simulink model "four_channel_bilateral_teleoperation_sampled"  (R2020b)
settings: Solver=VariableStepAuto  StartTime=0.0  StopTime=4.0  RelTol=1e-3
values from neighbouring files (symbols this model uses):
  A = 1    [four_channel_bilateral_teleoperation_kalman_params.m]    (also in four_channel_bilateral_teleoperation_params.m; kalman_test.m = [1 Ts Ts^2/2; 0 1 Ts; 0 0 1]; recursive_estimation.m = [1 Ts Ts^2/2; 0 1 Ts; 0 0 1]; scattering_based_bi_teleop_pf_kalman_params.m)
  Be = 100    [four_channel_bilateral_teleoperation_architecture_params.m]    (also in four_channel_bilateral_teleoperation_kalman_params.m = 0; four_channel_bilateral_teleoperation_params.m = 0; scattering_based_bi_teleop_pf_kalman_params.m = 10; scattering_based_bi_teleop_pf_params.m = 10)
  Bh = 70    [four_channel_bilateral_teleoperation_architecture_params.m]    (also in four_channel_bilateral_teleoperation_kalman_params.m; four_channel_bilateral_teleoperation_params.m; scattering_based_bi_teleop_pf_kalman_params.m = 1.5; scattering_based_bi_teleop_pf_params.m = 1.5)
  Bm = 1    [four_channel_bilateral_teleoperation_architecture_params.m]    (also in four_channel_bilateral_teleoperation_kalman_params.m = 0.8; four_channel_bilateral_teleoperation_params.m = 0.8; scattering_based_bi_teleop_pf_kalman_params.m = 0; scattering_based_bi_teleop_pp_kalman_params.m = 15)
  Bs = 1    [four_channel_bilateral_teleoperation_architecture_params.m]    (also in four_channel_bilateral_teleoperation_kalman_params.m = 3.2; four_channel_bilateral_teleoperation_params.m = 3.2; scattering_based_bi_teleop_pf_kalman_params.m = 40; scattering_based_bi_teleop_pf_params.m = 3)
  Dh = 500    [four_channel_bilateral_teleoperation_kalman_params.m]    (also in four_channel_bilateral_teleoperation_params.m = 100; scattering_based_bi_teleop_pf_kalman_params.m = 0; scattering_based_bi_teleop_pf_params.m = 17; scattering_based_bi_teleop_pp_kalman_params.m = 0)
  Dm = 5    [four_channel_bilateral_teleoperation_architecture_params.m]    (also in four_channel_bilateral_teleoperation_kalman_params.m = 0; four_channel_bilateral_teleoperation_params.m = 0; scattering_based_bi_teleop_pf_kalman_params.m = 0; scattering_based_bi_teleop_pf_params.m = 0)
  Ds = 10    [four_channel_bilateral_teleoperation_architecture_params.m]    (also in four_channel_bilateral_teleoperation_kalman_params.m = 0; four_channel_bilateral_teleoperation_params.m = 0; scattering_based_bi_teleop_pf_kalman_params.m = 0; scattering_based_bi_teleop_pf_params.m = 0)
  Fc = 1    [four_channel_bilateral_teleoperation_kalman_params.m]    (also in four_channel_bilateral_teleoperation_params.m; kalman_test.m = 10; scattering_based_bi_teleop_pf_kalman_params.m = 0.1; scattering_based_bi_teleop_pf_params.m)
  Fip = 1    [four_channel_bilateral_teleoperation_kalman_params.m]    (also in four_channel_bilateral_teleoperation_params.m; scattering_based_bi_teleop_pf_kalman_params.m = 5; scattering_based_bi_teleop_pf_params.m; scattering_based_bi_teleop_pp_kalman_params.m = 5)
  Je = 0    [four_channel_bilateral_teleoperation_architecture_params.m]    (also in four_channel_bilateral_teleoperation_kalman_params.m; four_channel_bilateral_teleoperation_params.m; scattering_based_bi_teleop_pf_kalman_params.m; scattering_based_bi_teleop_pf_params.m)
  Jh = 0.5    [four_channel_bilateral_teleoperation_architecture_params.m]    (also in four_channel_bilateral_teleoperation_kalman_params.m; four_channel_bilateral_teleoperation_params.m; scattering_based_bi_teleop_pf_kalman_params.m = 0; scattering_based_bi_teleop_pf_params.m = 0.05)
  Ke = 200    [four_channel_bilateral_teleoperation_architecture_params.m]    (also in four_channel_bilateral_teleoperation_kalman_params.m = 50; four_channel_bilateral_teleoperation_params.m; scattering_based_bi_teleop_pf_kalman_params.m; scattering_based_bi_teleop_pf_params.m)
  Kh = 2000    [four_channel_bilateral_teleoperation_architecture_params.m]    (also in four_channel_bilateral_teleoperation_kalman_params.m; four_channel_bilateral_teleoperation_params.m; scattering_based_bi_teleop_pf_kalman_params.m = 1; scattering_based_bi_teleop_pf_params.m = 0)
  Km = 1    [four_channel_bilateral_teleoperation_architecture_params.m]    (also in four_channel_bilateral_teleoperation_kalman_params.m; four_channel_bilateral_teleoperation_params.m; scattering_based_bi_teleop_pf_kalman_params.m = 0; scattering_based_bi_teleop_pp_kalman_params.m = 10)
  Ks = 1    [four_channel_bilateral_teleoperation_architecture_params.m]    (also in four_channel_bilateral_teleoperation_kalman_params.m = 4; four_channel_bilateral_teleoperation_params.m = 4; scattering_based_bi_teleop_pf_kalman_params.m = 50; scattering_based_bi_teleop_pf_params.m = 110)
  Mm = 0.5    [four_channel_bilateral_teleoperation_architecture_params.m]    (also in four_channel_bilateral_teleoperation_kalman_params.m; four_channel_bilateral_teleoperation_params.m; scattering_based_bi_teleop_pf_kalman_params.m; scattering_based_bi_teleop_pf_params.m)
  Ms = 2    [four_channel_bilateral_teleoperation_architecture_params.m]    (also in four_channel_bilateral_teleoperation_kalman_params.m; four_channel_bilateral_teleoperation_params.m; scattering_based_bi_teleop_pf_kalman_params.m; scattering_based_bi_teleop_pf_params.m)
  Ph = 2000    [four_channel_bilateral_teleoperation_kalman_params.m]    (also in four_channel_bilateral_teleoperation_params.m = 20100; scattering_based_bi_teleop_pf_kalman_params.m = 5; scattering_based_bi_teleop_pf_params.m = 23; scattering_based_bi_teleop_pp_kalman_params.m = 6)
  Ts = 0.001    [four_channel_bilateral_teleoperation_kalman_params.m]    (also in four_channel_bilateral_teleoperation_params.m; kalman_test.m; recursive_estimation.m; scattering_based_bi_teleop_pf_kalman_params.m)
undefined symbols (not defined in the file or in its folder): tau
libraries: simulink x4
settings Model: Creator=anuj  LastModifiedBy=filippo

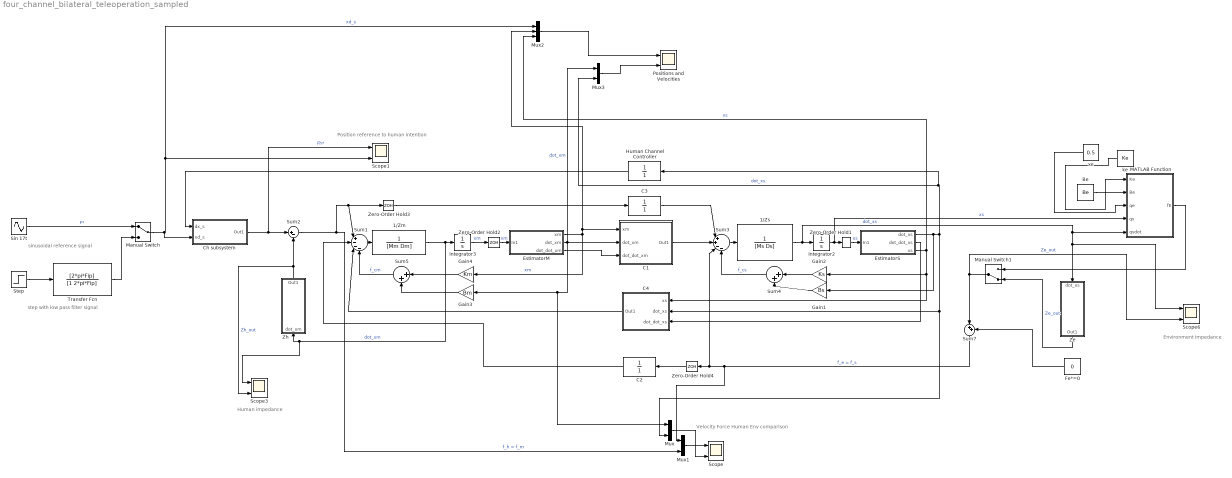
== system four_channel_bilateral_teleoperation_sampled ==
  note: Environment Impedance
  note: Human impedance
  note: Velocity Force Human Env comparison
  note: sinusoidal reference signal
  note: step with low pass filter signal
  note: Position reference to human intention
  1/Zm : TransferFcn  Denominator=[Mm Dm]
  1/Zs : TransferFcn  Denominator=[Ms Ds]
  Be : Constant  Value=Be
  C1 : Subsystem
  C2 : TransferFcn  Denominator=[1]
  C3 : TransferFcn  Denominator=[1]
  C4 : Subsystem
  Ch subsystem : Subsystem
  EstimatorM : Subsystem
  EstimatorS : Subsystem
  Fe*=0 : Constant  Value=0
  Gain1 : Gain  Gain=Bs
  Gain2 : Gain  Gain=Ks
  Gain3 : Gain  Gain=Bm
  Gain4 : Gain  Gain=Km
  Human Channel Controller : TransferFcn  Denominator=[1]
  Integrator2 : Integrator
  Integrator3 : Integrator
  MATLAB Function : MATLAB Function  TreatAsAtomicUnit=on
  Manual Switch : ManualSwitch
  Manual Switch1 : ManualSwitch  CurrentSetting=0
  Mux : Mux  Inputs=2
  Mux1 : Mux  Inputs=2
  Mux2 : Mux  Inputs=3
  Mux3 : Mux  Inputs=2
  Positions and Velocities : Scope  NumInputPorts=2
  Scope{,1,3,6} (4 alike) : Scope  NumInputPorts=2
  Sin 17t : Sin  Amplitude=A  Frequency=2*pi*Fc  SampleTime=0
  Step : Step  After=A  SampleTime=0
  Sum1 : Sum  Inputs=|+---
  Sum2 : Sum  Inputs=|+-
  Sum3 : Sum  Inputs=|++--
  Sum4 : Sum  Inputs=|++
  Sum5 : Sum  Inputs=|++
  Sum7 : Sum  Inputs=|++
  Transfer Fcn : TransferFcn  Numerator=[2*pi*Fip]  Denominator=[1 2*pi*Fip]
  Ze : Subsystem
  Zero-Order Hold{1..4} (4 alike) : ZeroOrderHold  SampleTime=Ts
  Zh : Subsystem
  ke : Constant  Value=Ke
  xe : Constant  Value=0.5
  wires:
  Mux/1 -> Scope/2
  Mux1/1 -> Scope/1
  Sum2/1 -> Zero-Order Hold3/1, Sum1/1, Mux1/2  "f_h = f_m"
  1/Zm/1 -> Scope3/1, Zh/1(dot_xm), Integrator3/1  "dot_xm"
  Sum1/1 -> 1/Zm/1
  C2/1 -> Sum1/2
  C3/1 -> Sum3/1
  Sum3/1 -> 1/Zs/1
  Fe*=0/1 -> Sum7/2
  Sum7/1 -> Mux1/1, Sum3/3, Zero-Order Hold4/1  "f_e = f_s"
  C4/1(Out1) -> Sum1/3
  Ch subsystem/1(Out1) -> Scope1/1, Sum2/1  "Fh*"
  Be/1 -> MATLAB Function/2(Be)
  xe/1 -> MATLAB Function/3(qe)
  ke/1 -> MATLAB Function/1(Ke)
  Transfer Fcn/1 -> Manual Switch/2
  Step/1 -> Transfer Fcn/1
  Human Channel Controller/1 -> Ch subsystem/1(dx_s)
  Manual Switch/1 -> Ch subsystem/2(xd_s), Mux2/1, Scope1/2  "xd_s"
  Sin 17t/1 -> Manual Switch/1  "F*"
  C1/1(Out1) -> Sum3/2
  MATLAB Function/1(fE) -> Manual Switch1/1
  Manual Switch1/1 -> Sum7/1, Scope6/2  "Ze_out"
  Zh/1(Out1) -> Scope3/2, Sum2/2  "Zh_out"
  Sum5/1 -> Sum1/4  "f_cm"
  Sum4/1 -> Sum3/4  "f_cs"
  Ze/1(Out1) -> Manual Switch1/2  "Ze_out"
  Mux2/1 -> Positions and Velocities/1
  Mux3/1 -> Positions and Velocities/2
  EstimatorS/1(dot_xs) -> Gain1/1, Mux/2, C4/2(dot_xs), Human Channel Controller/1, Mux3/2  "dot_xs"
  1/Zs/1 -> MATLAB Function/5(qsdot), Scope6/1, Ze/1(dot_xs), Integrator2/1  "dot_xs"
  Integrator2/1 -> Zero-Order Hold1/1, MATLAB Function/4(qs)  "xs"
  Gain2/1 -> Sum4/1
  Gain1/1 -> Sum4/2
  EstimatorS/3(xs) -> Mux2/3, Gain2/1, C4/1(xs)  "xs"
  Integrator3/1 -> Zero-Order Hold2/1  "xm"
  Gain4/1 -> Sum5/1
  Gain3/1 -> Sum5/2
  EstimatorM/2(dot_xm) -> Mux3/1, Mux/1, Gain3/1, C1/2(dot_xm)  "dot_xm"
  EstimatorS/2(dot_dot_xs) -> C4/3(dot_dot_xs)
  EstimatorM/3(dot_dot_xm) -> C1/3(dot_dot_xm)
  EstimatorM/1(xm) -> Mux2/2, C1/1(xm), Gain4/1  "xm"
  Zero-Order Hold1/1 -> EstimatorS/1(In1)  "xs"
  Zero-Order Hold2/1 -> EstimatorM/1(In1)  "xm"
  Zero-Order Hold3/1 -> C3/1
  Zero-Order Hold4/1 -> C2/1

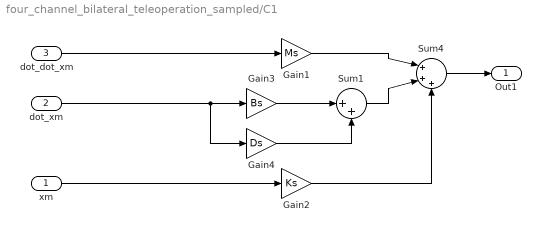
== system four_channel_bilateral_teleoperation_sampled/C1 ==
  xm : Inport
  dot_xm : Inport  Port=2
  dot_dot_xm : Inport  Port=3
  Gain1 : Gain  Gain=Ms
  Gain2 : Gain  Gain=Ks
  Gain3 : Gain  Gain=Bs
  Gain4 : Gain  Gain=Ds
  Sum1 : Sum  Inputs=|++
  Sum4 : Sum  Inputs=|+++
  Out1 : Outport
  wires:
  Sum4/1 -> Out1/1
  Gain1/1 -> Sum4/1
  xm/1 -> Gain2/1
  Gain2/1 -> Sum4/3
  Sum1/1 -> Sum4/2
  Gain4/1 -> Sum1/2
  Gain3/1 -> Sum1/1
  dot_dot_xm/1 -> Gain1/1
  dot_xm/1 -> Gain4/1, Gain3/1

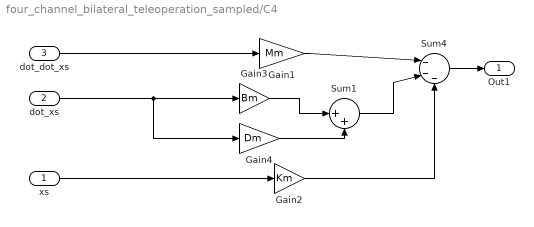
== system four_channel_bilateral_teleoperation_sampled/C4 ==
  xs : Inport
  dot_xs : Inport  Port=2
  dot_dot_xs : Inport  Port=3
  Gain1 : Gain  Gain=Mm
  Gain2 : Gain  Gain=Km
  Gain3 : Gain  Gain=Bm
  Gain4 : Gain  Gain=Dm
  Sum1 : Sum  Inputs=|++
  Sum4 : Sum  Inputs=|---
  Out1 : Outport
  wires:
  Sum4/1 -> Out1/1
  Gain1/1 -> Sum4/1
  xs/1 -> Gain2/1
  dot_xs/1 -> Gain3/1, Gain4/1
  Gain2/1 -> Sum4/3
  Sum1/1 -> Sum4/2
  Gain4/1 -> Sum1/2
  Gain3/1 -> Sum1/1
  dot_dot_xs/1 -> Gain1/1

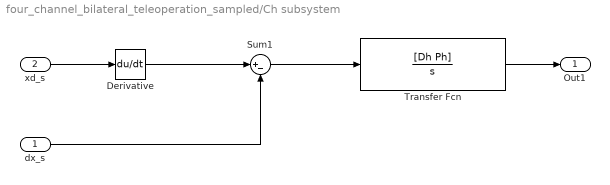
== system four_channel_bilateral_teleoperation_sampled/Ch subsystem ==
  dx_s : Inport
  xd_s : Inport  Port=2
  Derivative : Derivative
  Sum1 : Sum  Inputs=|+-
  Transfer Fcn : TransferFcn  Numerator=[Dh Ph]  Denominator=[1 0]
  Out1 : Outport
  wires:
  dx_s/1 -> Sum1/2
  Sum1/1 -> Transfer Fcn/1
  xd_s/1 -> Derivative/1
  Derivative/1 -> Sum1/1
  Transfer Fcn/1 -> Out1/1

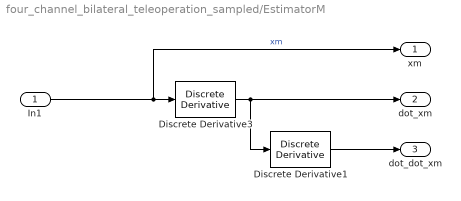
== system four_channel_bilateral_teleoperation_sampled/EstimatorM ==
  In1 : Inport
  Discrete Derivative1 : simulink/Discrete/Discrete Derivative  gainval=1.0  ICPrevScaledInput=0.0  OutMin=[]  OutMax=[]  OutDataType=fixdt(1, 16)  OutScaling=2^-10  DoSatur=off
  Discrete Derivative3 : simulink/Discrete/Discrete Derivative  gainval=1.0  ICPrevScaledInput=0.0  OutMin=[]  OutMax=[]  OutDataType=fixdt(1, 16)  OutScaling=2^-10  DoSatur=off
  xm : Outport
  dot_xm : Outport  Port=2
  dot_dot_xm : Outport  Port=3
  wires:
  Discrete Derivative3/1 -> Discrete Derivative1/1, dot_xm/1
  In1/1 -> xm/1, Discrete Derivative3/1  "xm"
  Discrete Derivative1/1 -> dot_dot_xm/1

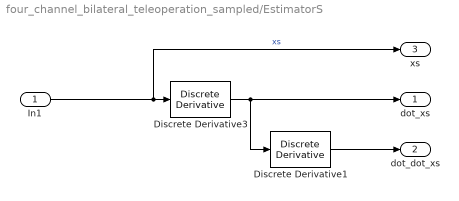
== system four_channel_bilateral_teleoperation_sampled/EstimatorS ==
  In1 : Inport
  Discrete Derivative1 : simulink/Discrete/Discrete Derivative  gainval=1.0  ICPrevScaledInput=0.0  OutMin=[]  OutMax=[]  OutDataType=fixdt(1, 16)  OutScaling=2^-10  DoSatur=off
  Discrete Derivative3 : simulink/Discrete/Discrete Derivative  gainval=1.0  ICPrevScaledInput=0.0  OutMin=[]  OutMax=[]  OutDataType=fixdt(1, 16)  OutScaling=2^-10  DoSatur=off
  dot_xs : Outport
  dot_dot_xs : Outport  Port=2
  xs : Outport  Port=3
  wires:
  Discrete Derivative3/1 -> Discrete Derivative1/1, dot_xs/1
  In1/1 -> xs/1, Discrete Derivative3/1  "xs"
  Discrete Derivative1/1 -> dot_dot_xs/1

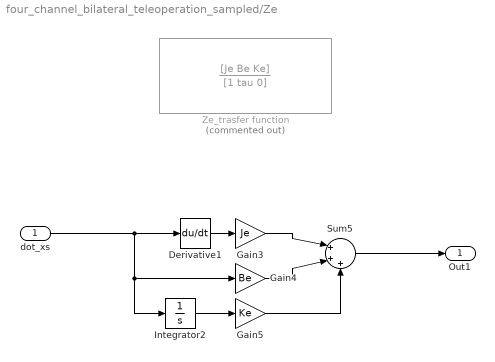
== system four_channel_bilateral_teleoperation_sampled/Ze ==
  dot_xs : Inport
  Derivative1 : Derivative
  Gain3 : Gain  Gain=Je
  Gain4 : Gain  Gain=Be
  Gain5 : Gain  Gain=Ke
  Integrator2 : Integrator
  Sum5 : Sum  Inputs=|+++
  Ze_trasfer function : TransferFcn  Commented=on  Numerator=[Je Be Ke]  Denominator=[1 tau 0]
  Out1 : Outport
  wires:
  Gain4/1 -> Sum5/2
  Gain3/1 -> Sum5/1
  Gain5/1 -> Sum5/3
  Sum5/1 -> Out1/1
  Integrator2/1 -> Gain5/1
  dot_xs/1 -> Integrator2/1, Gain4/1, Derivative1/1
  Derivative1/1 -> Gain3/1

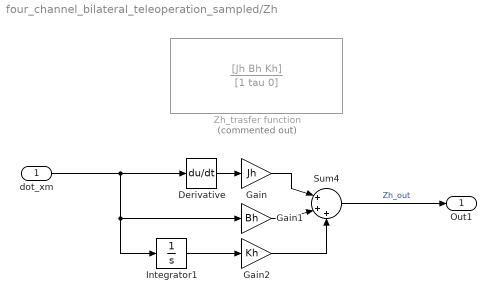
== system four_channel_bilateral_teleoperation_sampled/Zh ==
  dot_xm : Inport
  Derivative : Derivative
  Gain : Gain  Gain=Jh
  Gain1 : Gain  Gain=Bh
  Gain2 : Gain  Gain=Kh
  Integrator1 : Integrator
  Sum4 : Sum  Inputs=|+++
  Zh_trasfer function : TransferFcn  Commented=on  Numerator=[Jh Bh Kh]  Denominator=[1 tau 0]
  Out1 : Outport
  wires:
  Derivative/1 -> Gain/1
  Integrator1/1 -> Gain2/1
  Gain2/1 -> Sum4/3
  Gain1/1 -> Sum4/2
  Gain/1 -> Sum4/1
  Sum4/1 -> Out1/1  "Zh_out"
  dot_xm/1 -> Gain1/1, Integrator1/1, Derivative/1

== matlab function four_channel_bilateral_teleoperation_sampled/MATLAB Function ==
  data: Ke input; fE output; Be input; qe input; qs input; qsdot input
function fE = environment(Ke, Be, qe, qs, qsdot)
    if qs > qe
        fE = Ke * (qs - qe) + Be * qsdot;
    else
        fE = 0;
    end
end
